simulink model "Prob6_ReferenceModel"  (R2020b)
settings: Solver=FixedStepAuto  StartTime=0.0  StopTime=10.0  FixedStep=0.2  RelTol=1e-3
settings Model: Creator=admin  LastModifiedBy=admin
settings DataIOCC: SaveOutput=off  SaveTime=off

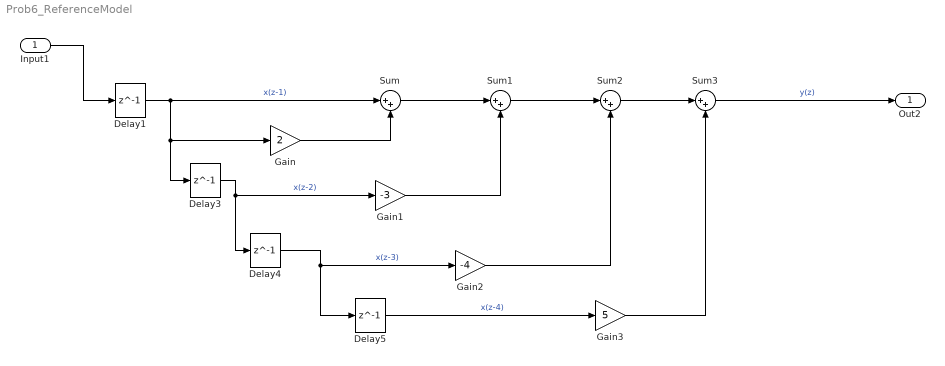
== system Prob6_ReferenceModel ==
  Input1 : Inport  OutDataTypeStr=double  PortDimensions=1  SampleTime=[0.20000000000000001,0]
  Delay{1,3..5} (4 alike) : Delay  DelayLength=1
  Gain : Gain  Gain=2
  Gain1 : Gain  Gain=-3
  Gain2 : Gain  Gain=-4
  Gain3 : Gain  Gain=5
  Sum{,1..3} (4 alike) : Sum  Inputs=|++
  Out2 : Outport  OutDataTypeStr=double  PortDimensions=1  SampleTime=[0.20000000000000001,0]
  wires:
  Delay4/1 -> Gain2/1, Delay5/1  "x(z-3)"
  Delay3/1 -> Gain1/1, Delay4/1  "x(z-2)"
  Sum1/1 -> Sum2/1
  Sum/1 -> Sum1/1
  Sum3/1 -> Out2/1  "y(z)"
  Gain3/1 -> Sum3/2
  Delay5/1 -> Gain3/1  "x(z-4)"
  Gain2/1 -> Sum2/2
  Input1/1 -> Delay1/1
  Gain/1 -> Sum/2
  Delay1/1 -> Sum/1, Gain/1, Delay3/1  "x(z-1)"
  Gain1/1 -> Sum1/2
  Sum2/1 -> Sum3/1
